simulink model "LaRegulationDUnSystemDePremier"  (R2017a)
settings: Solver=VariableStepAuto  StartTime=0.0  StopTime=10.0  RelTol=1e-3
values from neighbouring files (symbols this model uses):
  K1 = 1    [declaration_des_variables.m]
  K2 = 10    [declaration_des_variables.m]
  K3 = 100    [declaration_des_variables.m]
  K4 = 1000    [declaration_des_variables.m]
settings Model: Creator=PC  LastModifiedBy=PC

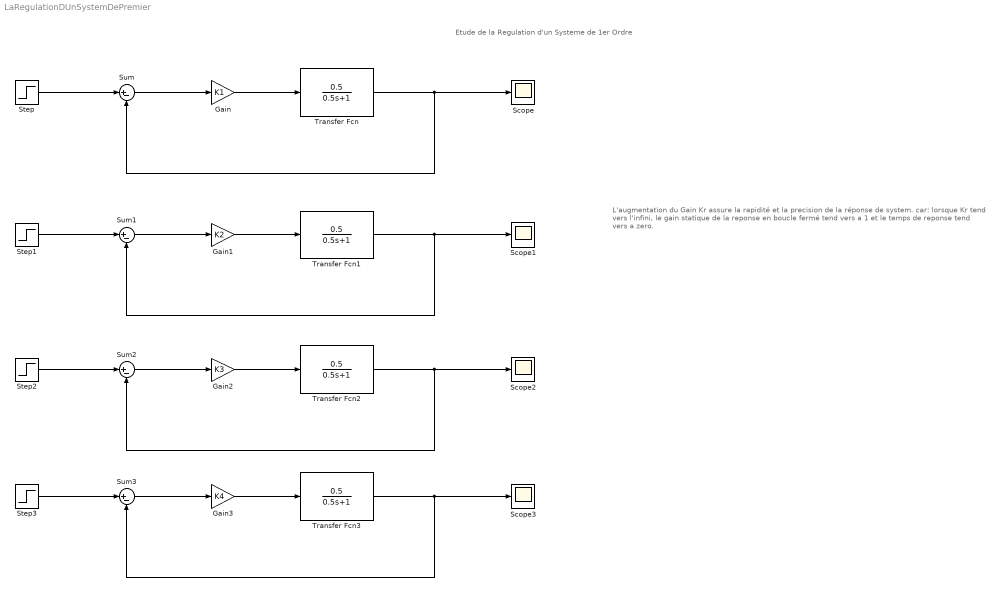
== system LaRegulationDUnSystemDePremier ==
  note: L'augmentation du Gain Kr assure la rapidité et la precision de la réponse de system.
      |
      | car: lorsque Kr tend vers l'infini, le gain statique de la reponse en boucle fermé tend vers a 1 et le temps de reponse tend vers a zero.
  note: Etude de la Regulation d'un Systeme de 1er Ordre
  Gain : Gain  Gain=K1
  Gain1 : Gain  Gain=K2
  Gain2 : Gain  Gain=K3
  Gain3 : Gain  Gain=K4
  Scope{,1..3} (4 alike) : Scope
  Step{,1..3} (4 alike) : Step  SampleTime=0
  Sum{,1..3} (4 alike) : Sum  Inputs=|+-
  Transfer Fcn{,1..3} (4 alike) : TransferFcn  Numerator=[0.5]  Denominator=[0.5 1]
  wires:
  Sum/1 -> Gain/1
  Transfer Fcn/1 -> Sum/2, Scope/1
  Step/1 -> Sum/1
  Gain/1 -> Transfer Fcn/1
  Gain1/1 -> Transfer Fcn1/1
  Step1/1 -> Sum1/1
  Transfer Fcn1/1 -> Scope1/1, Sum1/2
  Sum1/1 -> Gain1/1
  Sum2/1 -> Gain2/1
  Transfer Fcn2/1 -> Sum2/2, Scope2/1
  Step2/1 -> Sum2/1
  Gain2/1 -> Transfer Fcn2/1
  Gain3/1 -> Transfer Fcn3/1
  Step3/1 -> Sum3/1
  Transfer Fcn3/1 -> Scope3/1, Sum3/2
  Sum3/1 -> Gain3/1
